simulink model "VectorMux"  (Simulink 7.4)
settings: Solver=VariableStepDiscrete  StartTime=0.0  StopTime=10.0  MaxStep=1  RelTol=1e-3
libraries: BLOM_Lib x3
settings Model: Creator=Tony  LastModifiedBy=Tony
settings DataIOCC: SaveOutput=off  SaveTime=off
settings DebuggingCC: StrictBusMsg=ErrorLevel1

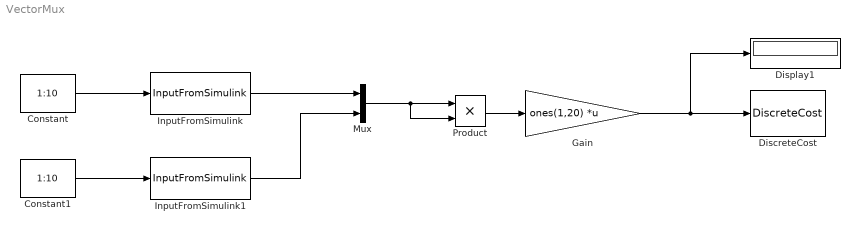
== system VectorMux ==
  Constant : Constant  Value=1:10  SampleTime=1
  Constant1 : Constant  Value=1:10  SampleTime=1
  DiscreteCost : BLOM_Lib/DiscreteCost  SystemSampleTime=-1  initial_step=on  final_step=on  intermediate_step=on
  Display1 : Display
  Gain : Gain  Gain=ones(1,20)  Multiplication=Matrix(K*u)
  InputFromSimulink : BLOM_Lib/InputFromSimulink  SystemSampleTime=-1  interpType=Zero-Order Hold
  InputFromSimulink1 : BLOM_Lib/InputFromSimulink  SystemSampleTime=-1  interpType=Zero-Order Hold
  Mux : Mux  Inputs=2
  Product : Product  RndMeth=Zero
  wires:
  Constant/1 -> InputFromSimulink/1
  Constant1/1 -> InputFromSimulink1/1
  InputFromSimulink/1 -> Mux/1
  InputFromSimulink1/1 -> Mux/2
  Mux/1 -> Product/1, Product/2
  Product/1 -> Gain/1
  Gain/1 -> Display1/1, DiscreteCost/1
